simulink model "HSVmodel"  (R2023b)
settings: Solver=ode3  StartTime=0.0  StopTime=50.0  FixedStep=0.02  RelTol=1e-3  EnableMultiTasking=on
InitFcn:
  | Init_AeroSpaceBlk
settings Model: Creator=think  LastModifiedBy=asus
settings SolverCC: AlgebraicLoopSolver=TrustRegion
settings DataIOCC: LimitDataPoints=on  SaveFormat=Array  SignalLoggingSaveFormat=ModelDataLogs  ReturnWorkspaceOutputs=off
settings OptimizationCC: ExpressionDepthLimit=2147483647  InitFltsAndDblsToZero=on  LifeSpan=inf
settings DebuggingCC: SaveWithParameterizedLinksMsg=none  UnderspecifiedInitializationDetection=Classic  MergeDetectMultiDrivingBlocksExec=none  SignalResolutionControl=TryResolveAllWithWarning  MultiTaskDSMMsg=warning  MultiTaskCondExecSysMsg=none  FcnCallInpInsideContextMsg=warning  UnconnectedInputMsg=warning  UnconnectedOutputMsg=warning  UnconnectedLineMsg=warning  StateNameClashWarn=warning  SFUnexpectedBacktrackingDiag=warning  SFNoUnconditionalDefaultTransitionDiag=warning  SFExecutionAtInitializationDiag=none  ArithmeticOperatorsInVariantConditions=warning
settings HardwareCC: ProdBitPerPointer=32  ProdBitPerSizeT=32  ProdBitPerPtrDiffT=32  ProdLargestAtomicFloat=None  ProdIntDivRoundTo=Undefined  ProdEndianess=Unspecified  ProdWordSize=32  ProdHWDeviceType=32-bit Generic
settings ModelReferenceCC: PropagateSignalLabelsOutOfModel=off
settings SFSimCC: SimUseLocalCustomCode=off  CustomCodeUndefinedFunction=UseInterfaceOnly
settings RTWCC: RTWUseLocalCustomCode=off
settings CodeAppCC: StateflowObjectComments=on
settings GRTTargetCC: TargetFcnLib=ansi_tfl_tmw.mat  TargetLangStandard=C89/C90 (ANSI)  CombineOutputUpdateFcns=off  GRTInterface=on
settings ConfigComp: CovMetricSettings=dw  CovSaveCumulativeToWorkspaceVar=on  CovSaveSingleToWorkspaceVar=on  CovExternalEMLEnable=off  CovSFcnEnable=off

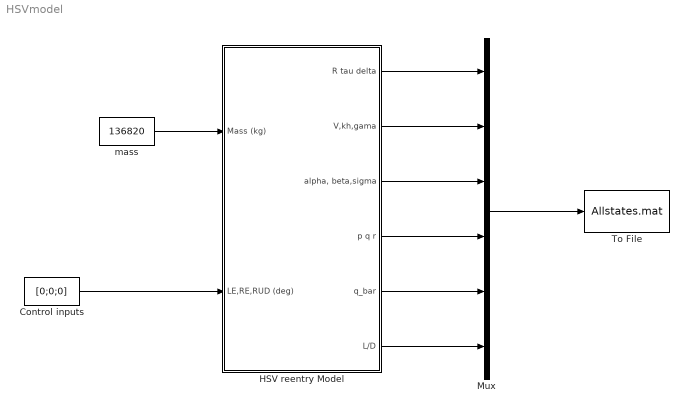
== system HSVmodel ==
  Control inputs : Constant  Value=[0;0;0]
  HSV reentry Model : Subsystem
  Mux : Mux  Inputs=6
  To File : ToFile  Filename=Allstates.mat  MatrixName=Allstates
  "mass " : Constant  Value=136820
  wires:
  "mass "/1 -> HSV reentry Model/1(Mass (kg))
  Control inputs/1 -> HSV reentry Model/2(LE,RE,RUD (deg))
  HSV reentry Model/1(R tau delta) -> Mux/1
  HSV reentry Model/2(V,kh,gama) -> Mux/2
  HSV reentry Model/3("alpha, beta,sigma") -> Mux/3
  HSV reentry Model/4(p q r) -> Mux/4
  Mux/1 -> To File/1
  HSV reentry Model/5(q_bar) -> Mux/5
  HSV reentry Model/6(L/D) -> Mux/6

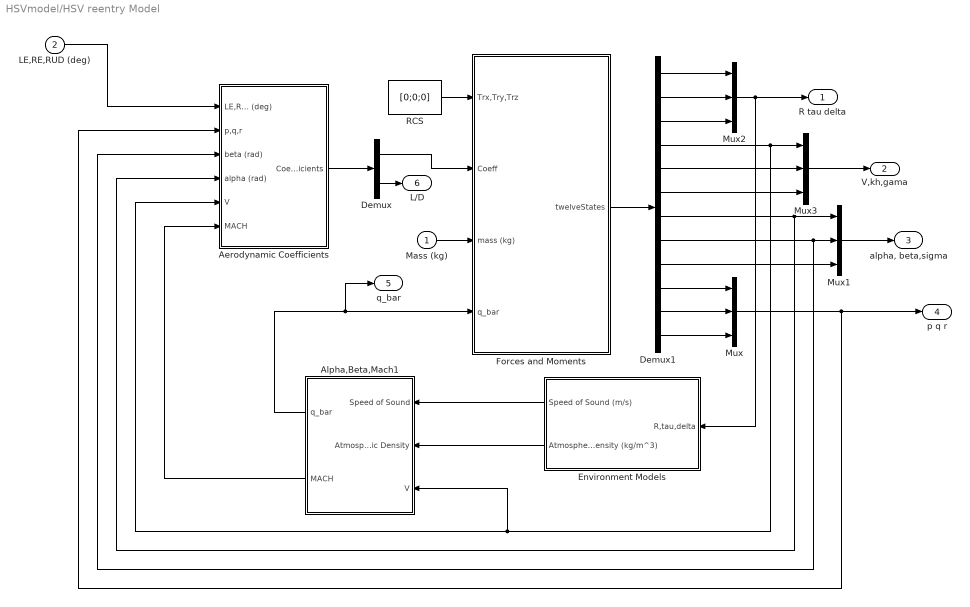
== system HSVmodel/HSV reentry Model ==
  Mass (kg) : Inport
  LE,RE,RUD (deg) : Inport  Port=2
  Aerodynamic Coefficients : Subsystem
  Alpha,Beta,Mach1 : Subsystem
  Demux : Demux  Outputs=[6;1]
  Demux1 : Demux  Outputs=12
  Environment Models : Subsystem
  Forces and Moments : Subsystem
  Mux{,1..3} (4 alike) : Mux  Inputs=3
  RCS : Constant  Value=[0;0;0]
  R tau delta : Outport  InitialOutput=0
  V,kh,gama : Outport  Port=2  InitialOutput=0
  "alpha, beta,sigma" : Outport  Port=3  InitialOutput=0
  p q r : Outport  Port=4  InitialOutput=0
  q_bar : Outport  Port=5  InitialOutput=0
  L/D : Outport  Port=6  InitialOutput=0
  wires:
  LE,RE,RUD (deg)/1 -> Aerodynamic Coefficients/1(LE,RE,RUD (deg))
  Alpha,Beta,Mach1/2(MACH) -> Aerodynamic Coefficients/6(MACH)
  Mass (kg)/1 -> Forces and Moments/3(mass (kg))
  Alpha,Beta,Mach1/1(q_bar) -> Forces and Moments/4(q_bar), q_bar/1
  Mux2/1 -> R tau delta/1, Environment Models/1(R,tau,delta)
  RCS/1 -> Forces and Moments/1(Trx,Try,Trz)
  Mux1/1 -> "alpha, beta,sigma"/1
  Mux3/1 -> V,kh,gama/1
  Mux/1 -> p q r/1, Aerodynamic Coefficients/2(p,q,r)
  Environment Models/1(Speed of Sound (m/s)) -> Alpha,Beta,Mach1/1(Speed of Sound)
  Environment Models/2(Atmospheric Density (kg/m^3)) -> Alpha,Beta,Mach1/2(Atmospheric Density)
  Forces and Moments/1(twelveStates) -> Demux1/1
  Demux1/1 -> Mux2/1
  Demux1/2 -> Mux2/2
  Demux1/3 -> Mux2/3
  Demux1/4 -> Mux3/1, Aerodynamic Coefficients/5(V), Alpha,Beta,Mach1/3(V)
  Demux1/5 -> Mux3/2
  Demux1/6 -> Mux3/3
  Demux1/7 -> Mux1/1, Aerodynamic Coefficients/4(alpha (rad))
  Demux1/8 -> Aerodynamic Coefficients/3(beta (rad)), Mux1/2
  Demux1/9 -> Mux1/3
  Demux1/10 -> Mux/1
  Demux1/11 -> Mux/2
  Demux1/12 -> Mux/3
  Aerodynamic Coefficients/1(Coefficients) -> Demux/1
  Demux/1 -> Forces and Moments/2(Coeff)
  Demux/2 -> L/D/1

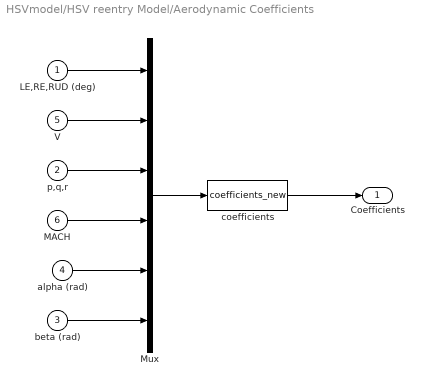
== system HSVmodel/HSV reentry Model/Aerodynamic Coefficients ==
  LE,RE,RUD (deg) : Inport
  p,q,r : Inport  Port=2
  beta (rad) : Inport  Port=3
  alpha (rad) : Inport  Port=4
  V : Inport  Port=5  PortDimensions=1
  MACH : Inport  Port=6
  Mux : Mux  Inputs=6
  coefficients : MATLABFcn  MATLABFcn=coefficients_new  OutputDimensions=7  Output1D=off
  Coefficients : Outport  InitialOutput=0
  wires:
  alpha (rad)/1 -> Mux/5
  V/1 -> Mux/2
  p,q,r/1 -> Mux/3
  MACH/1 -> Mux/4
  Mux/1 -> coefficients/1
  coefficients/1 -> Coefficients/1
  LE,RE,RUD (deg)/1 -> Mux/1
  beta (rad)/1 -> Mux/6

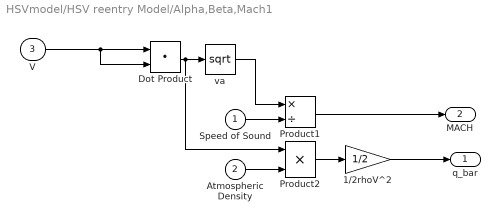
== system HSVmodel/HSV reentry Model/Alpha,Beta,Mach1 ==
  Speed of Sound : Inport
  Atmospheric Density : Inport  Port=2
  V : Inport  Port=3  PortDimensions=1
  1/2rhoV^2 : Gain  Gain=1/2  SaturateOnIntegerOverflow=on  OutDataTypeStr=Inherit: Same as input  ParamDataTypeStr=Inherit: Same as input
  Dot Product : DotProduct  OutDataTypeStr=Inherit: Inherit via internal rule
  Product1 : Product  Inputs=*/  InputSameDT=on  SaturateOnIntegerOverflow=on  OutDataTypeStr=Inherit: Same as first input
  Product2 : Product  InputSameDT=on  SaturateOnIntegerOverflow=on  OutDataTypeStr=Inherit: Same as first input
  va : Math  Operator=sqrt  SignedPower=on
  q_bar : Outport  InitialOutput=0
  MACH : Outport  Port=2
  wires:
  1/2rhoV^2/1 -> q_bar/1
  Product2/1 -> 1/2rhoV^2/1
  Atmospheric Density/1 -> Product2/2
  Dot Product/1 -> va/1, Product2/1
  Product1/1 -> MACH/1
  va/1 -> Product1/1
  Speed of Sound/1 -> Product1/2
  V/1 -> Dot Product/2, Dot Product/1

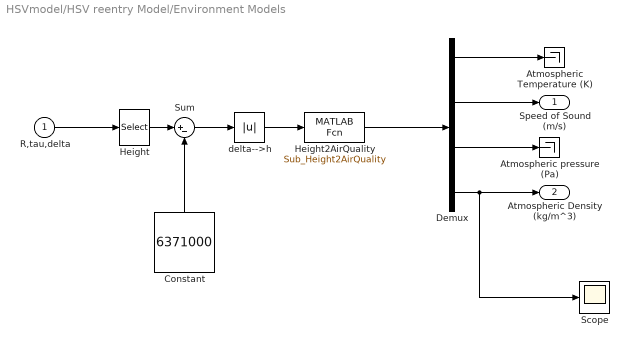
== system HSVmodel/HSV reentry Model/Environment Models ==
  R,tau,delta : Inport  PortDimensions=3
  Atmospheric Temperature (K) : Terminator
  Atmospheric pressure (Pa) : Terminator
  Constant : Constant  Value=6371000
  Demux : Demux
      settings: DisplayOption=none
  Height : Selector  InputPortWidth=3  IndexOptions=Index vector (dialog)  Indices=[1]  OutputSizes=1
  Height2AirQuality : MATLABFcn  MATLABFcn=Sub_Height2AirQuality  OutputDimensions=4  OutputSignalType=real  Output1D=off
  Scope : Scope
  Sum : Sum  Inputs=|+-
  delta-->h : Abs
  Speed of Sound (m/s) : Outport
  Atmospheric Density (kg/m^3) : Outport  Port=2
  wires:
  delta-->h/1 -> Height2AirQuality/1
  Demux/1 -> Atmospheric Temperature (K)/1
  Demux/2 -> Speed of Sound (m/s)/1
  Demux/3 -> Atmospheric pressure (Pa)/1
  Demux/4 -> Atmospheric Density (kg/m^3)/1, Scope/1
  Height2AirQuality/1 -> Demux/1
  Constant/1 -> Sum/2
  R,tau,delta/1 -> Height/1
  Height/1 -> Sum/1
  Sum/1 -> delta-->h/1

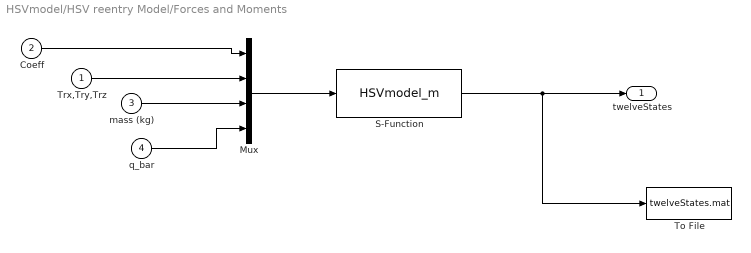
== system HSVmodel/HSV reentry Model/Forces and Moments ==
  Trx,Try,Trz : Inport
  Coeff : Inport  Port=2
  mass (kg) : Inport  Port=3
  q_bar : Inport  Port=4
  Mux : Mux
  S-Function : S-Function  FunctionName=HSVmodel_m  SFunctionDeploymentMode=off  EnableBusSupport=off
  To File : ToFile  Filename=twelveStates.mat  MatrixName=twelveStates
  twelveStates : Outport
  wires:
  Coeff/1 -> Mux/1
  q_bar/1 -> Mux/4
  Trx,Try,Trz/1 -> Mux/2
  mass (kg)/1 -> Mux/3
  Mux/1 -> S-Function/1
  S-Function/1 -> To File/1, twelveStates/1
